simulink model "wheel_orientation_estimation"  (R2020a)
settings: Solver=FixedStepAuto  StartTime=0.0  StopTime=30  FixedStep=1e-3  RelTol=1e-3
libraries: dspstat3 x4, dspfdesign x2, simulink x1, dspsrcs4 x1
settings Model: Creator=nils_  LastModifiedBy=nils_

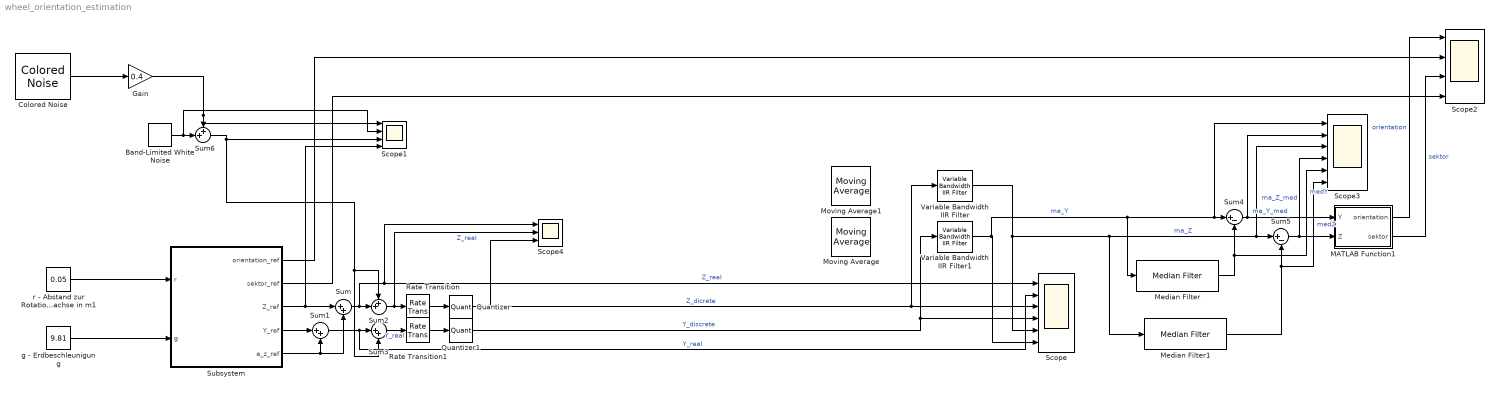
== system wheel_orientation_estimation ==
  Band-Limited White Noise : simulink/Sources/Band-Limited White Noise  Cov=[0.00001]  Ts=1e-3  seed=[23341]
  Colored Noise : dspsrcs4/Colored Noise  Color=pink  InverseFrequencyPower=1  BoundedOutput=off  NumChannels=1  OutputDataType=double  SamplesPerFrame=1  SampleTime=1/100  RandomStream=mt19937ar with seed  Seed=67  SimulateUsing=Interpreted execution
      settings: SourceProductBaseCode=DS
  Gain : Gain  Gain=0.4
  MATLAB Function1 : MATLAB Function  TreatAsAtomicUnit=on
  Median Filter : dspstat3/Median Filter  WindowLength=14  SimulateUsing=Interpreted execution
      settings: SourceProductBaseCode=DS
  Median Filter1 : dspstat3/Median Filter  WindowLength=14  SimulateUsing=Interpreted execution
      settings: SourceProductBaseCode=DS
  Moving Average : dspstat3/Moving Average  Method=Sliding window  ForgettingFactorPort=off  SpecifyWindowLength=on  WindowLength=7  ForgettingFactor=0.9  SimulateUsing=Code generation
  Moving Average1 : dspstat3/Moving Average  Method=Sliding window  ForgettingFactorPort=off  SpecifyWindowLength=on  WindowLength=7  ForgettingFactor=0.9  SimulateUsing=Code generation
  Quantizer : Quantizer  QuantizationInterval=(16/1024)/2
  Quantizer1 : Quantizer  QuantizationInterval=(16/1024)/2
  Rate Transition : RateTransition  OutPortSampleTime=1/100
  Rate Transition1 : RateTransition  OutPortSampleTime=1/100
  Scope : Scope  NumInputPorts=6
  Scope1 : Scope  NumInputPorts=4
  Scope2 : Scope  NumInputPorts=4
  Scope3 : Scope  NumInputPorts=6
  Scope4 : Scope  NumInputPorts=3
  Subsystem : Subsystem
  Sum : Sum  Inputs=|++
  Sum1 : Sum  Inputs=|++
  Sum2 : Sum  Inputs=++|
  Sum3 : Sum  Inputs=|++
  Sum4 : Sum  Inputs=|+-
  Sum5 : Sum  Inputs=|+-
  Sum6 : Sum  Inputs=++|
  Variable Bandwidth IIR Filter : dspfdesign/Variable Bandwidth IIR Filter  FilterType=Lowpass  FilterOrder=1  PassbandFrequencyPort=off  PassbandFrequency=10  CenterFrequencyPort=off  CenterFrequency=44100/4  BandwidthPort=off  Bandwidth=7680  PassbandRipple=1  StopbandAttenuation=60  InheritSampleRate=on  SampleRate=44100  SimulateUsing=Code generation
      settings: SourceProductBaseCode=DS
  Variable Bandwidth IIR Filter1 : dspfdesign/Variable Bandwidth IIR Filter  FilterType=Lowpass  FilterOrder=1  PassbandFrequencyPort=off  PassbandFrequency=10  CenterFrequencyPort=off  CenterFrequency=44100/4  BandwidthPort=off  Bandwidth=7680  PassbandRipple=1  StopbandAttenuation=60  InheritSampleRate=on  SampleRate=44100  SimulateUsing=Code generation
      settings: SourceProductBaseCode=DS
  g - Erdbeschleunigung : Constant  Value=9.81
  r - Abstand zur Rotationsachse in m1 : Constant  Value=0.05
  wires:
  Subsystem/3(Z_ref) -> Scope1/4, Sum/1
  Subsystem/5(a_z_ref) -> Sum1/2, Sum/2
  Subsystem/4(Y_ref) -> Sum1/1
  Sum3/1 -> Rate Transition1/1  "Y_real"
  Sum2/1 -> Scope4/2, Rate Transition/1  "Z_real"
  Quantizer/1 -> Scope4/3, Variable Bandwidth IIR Filter/1, Scope/3  "Z_dicrete"
  Quantizer1/1 -> Variable Bandwidth IIR Filter1/1, Scope/4  "Y_discrete"
  Rate Transition/1 -> Quantizer/1
  Rate Transition1/1 -> Quantizer1/1
  Sum6/1 -> Sum3/2, Sum2/1, Scope1/3
  Sum/1 -> Scope4/1, Scope/1, Sum2/2  "Z_real"
  Sum1/1 -> Scope/2, Sum3/1  "Y_real"
  MATLAB Function1/1(orientation) -> Scope2/1  "orientation"
  MATLAB Function1/2(sektor) -> Scope2/3  "sektor"
  Sum4/1 -> MATLAB Function1/1(Y), Scope3/2  "ma_Y_med"
  Sum5/1 -> MATLAB Function1/2(Z), Scope3/4  "ma_Z_med"
  Subsystem/1(orientation_ref) -> Scope2/2
  Subsystem/2(sektor_ref) -> Scope2/4
  Median Filter/1 -> Scope3/5, Sum4/2  "medY"
  Median Filter1/1 -> Scope3/6, Sum5/2  "medZ"
  g - Erdbeschleunigung/1 -> Subsystem/2(g)
  r - Abstand zur Rotationsachse in m1/1 -> Subsystem/1(r)
  Band-Limited White Noise/1 -> Scope1/2, Sum6/2
  Colored Noise/1 -> Gain/1
  Gain/1 -> Scope1/1, Sum6/1
  Variable Bandwidth IIR Filter1/1 -> Median Filter/1, Scope3/1, Sum4/1, Scope/6  "ma_Y"
  Variable Bandwidth IIR Filter/1 -> Median Filter1/1, Sum5/1, Scope3/3, Scope/5  "ma_Z"

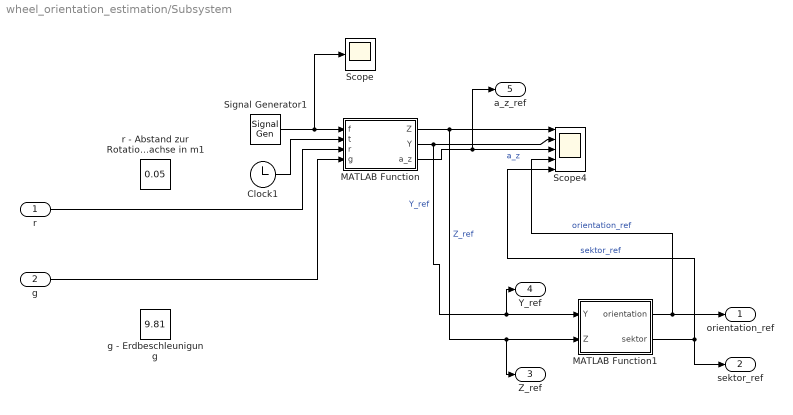
== system wheel_orientation_estimation/Subsystem ==
  r : Inport
  g : Inport  Port=2
  Clock1 : Clock
  MATLAB Function : MATLAB Function  TreatAsAtomicUnit=on
  MATLAB Function1 : MATLAB Function  TreatAsAtomicUnit=on
  Scope : Scope
  Scope4 : Scope  NumInputPorts=5
  Signal Generator1 : SignalGenerator  Amplitude=8  Frequency=0.25/30
  g - Erdbeschleunigung : Constant  Value=9.81
  r - Abstand zur Rotationsachse in m1 : Constant  Value=0.05
  orientation_ref : Outport
  sektor_ref : Outport  Port=2
  Z_ref : Outport  Port=3
  Y_ref : Outport  Port=4
  a_z_ref : Outport  Port=5
  wires:
  MATLAB Function1/1(orientation) -> orientation_ref/1, Scope4/4  "orientation_ref"
  MATLAB Function/3(a_z) -> a_z_ref/1, Scope4/3  "a_z"
  MATLAB Function/1(Z) -> Z_ref/1, MATLAB Function1/2(Z), Scope4/1  "Z_ref"
  g/1 -> MATLAB Function/4(g)
  MATLAB Function/2(Y) -> Y_ref/1, MATLAB Function1/1(Y), Scope4/2  "Y_ref"
  r/1 -> MATLAB Function/3(r)
  Clock1/1 -> MATLAB Function/2(t)
  Signal Generator1/1 -> Scope/1, MATLAB Function/1(f)
  MATLAB Function1/2(sektor) -> sektor_ref/1, Scope4/5  "sektor_ref"

== matlab function wheel_orientation_estimation/Subsystem/MATLAB Function1 ==
  data: Y input; orientation output; Z input; sektor output
function [orientation,sektor] = fcn(Y,Z)

orientation = 10;
sektor = 0;

% if ((Y>0)==1)==((Z>=0)==1) % I
%     orientation = atan(Z/Y);
%     sektor = 1;
% elseif ((Y<=0)==1)==((Z>0)==1)   % II
%     orientation = (pi/2)+atan(-Y/Z);
%     sektor = 2;
% elseif ((Z<=0)==1)==((Y<0)==1)    % III
%     orientation = pi+atan(Z/Y);
%     sektor = 3;
% elseif ((Y>=0)==1)==((Z<0)==1)    % IV
%     orientation = (pi*3/2)+atan(Y/-Z);
%     sektor = 4;
% else
%     orientation = 10;
%     sektor = 0;
% end

if Y>0
    if Z>=0 % I
        orientation = atan(Z/Y);
        sektor = 1;  
    end
end

if Y<=0
    if Z>=0 % II
        orientation = (pi/2)+atan(-Y/Z);
        sektor = 2;
    end
end

if Z<=0
    if Y<0  % III
        orientation = pi+atan(Z/Y);
        sektor = 3;
    end
end

if Y>=0
    if Z<0  % IV
        orientation = (pi*3/2)+atan(Y/-Z);
        sektor = 4;
    end
end

== matlab function wheel_orientation_estimation/Subsystem/MATLAB Function ==
  data: f input; Z output; t input; Y output; a_z output; r input; g input
function [Z,Y,a_z] = fcn(f,t,r,g)

a_z = ((2*pi*f)*(2*pi*f)*r)/g;
Y = sin(2*pi*f*t);
Z = cos(2*pi*f*t);

== matlab function wheel_orientation_estimation/MATLAB Function1 ==
  data: Y input; orientation output; Z input; sektor output
function [orientation,sektor] = fcn(Y,Z)

orientation = 10;
sektor = 0;

% if ((Y>0)==1)==((Z>=0)==1) % I
%     orientation = atan(Z/Y);
%     sektor = 1;
% elseif ((Y<=0)==1)==((Z>0)==1)   % II
%     orientation = (pi/2)+atan(-Y/Z);
%     sektor = 2;
% elseif ((Z<=0)==1)==((Y<0)==1)    % III
%     orientation = pi+atan(Z/Y);
%     sektor = 3;
% elseif ((Y>=0)==1)==((Z<0)==1)    % IV
%     orientation = (pi*3/2)+atan(Y/-Z);
%     sektor = 4;
% else
%     orientation = 10;
%     sektor = 0;
% end

if Y>0
    if Z>=0 % I
        orientation = atan(Z/Y);
        sektor = 1;  
    end
end

if Y<=0
    if Z>=0 % II
        orientation = (pi/2)+atan(-Y/Z);
        sektor = 2;
    end
end

if Z<=0
    if Y<0  % III
        orientation = pi+atan(Z/Y);
        sektor = 3;
    end
end

if Y>=0
    if Z<0  % IV
        orientation = (pi*3/2)+atan(Y/-Z);
        sektor = 4;
    end
end
